simulink subsystem "SchlittenVorsteuerung"  (R2020a)
settings: Solver=VariableStepAuto  StartTime=0.0  StopTime=10.0  RelTol=1e-3
model mask{SP=simparams.gesamtmodell.schlittenpendel, vorst=simparams.vorst}
  mask prompts: SP "Schlitten Parameter"; vorst "Vorsteuerung"
undefined symbols (not defined in the file or in its folder): d0, Fc0, M, vorstC, vorstD, x0_p_c076_vorst
settings Model: Creator=Tobias  LastModifiedBy=Tobias

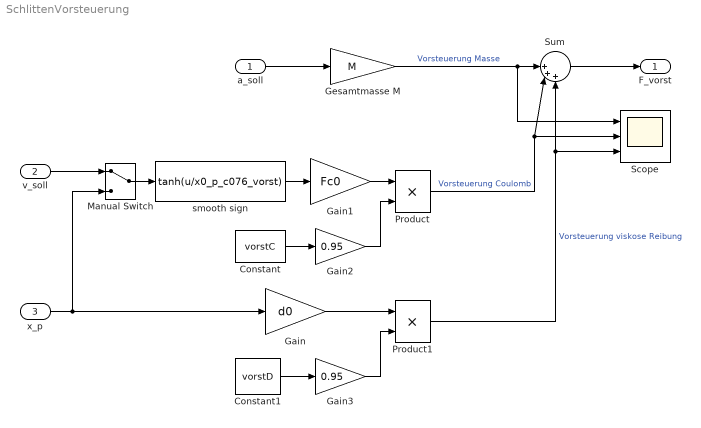
== system SchlittenVorsteuerung ==
  a_soll : Inport
  v_soll : Inport  Port=2
  x_p : Inport  Port=3
  Constant : Constant  Value=vorstC
  Constant1 : Constant  Value=vorstD
  Gain : Gain  Gain=d0
  Gain1 : Gain  Gain=Fc0
  Gain2 : Gain  Gain=0.95
  Gain3 : Gain  Gain=0.95
  Gesamtmasse M : Gain  Gain=M
  Manual Switch : ManualSwitch
  Product : Product  RndMeth=Zero
  Product1 : Product  RndMeth=Zero
  Scope : Scope  NumInputPorts=3
  Sum : Sum  Inputs=||+++
  smooth sign : Fcn  Expr=tanh(u/x0_p_c076_vorst)
  F_vorst : Outport
  wires:
  Constant1/1 -> Gain3/1
  Gain/1 -> Product1/1
  Product1/1 -> Scope/3, Sum/3  "Vorsteuerung viskose Reibung"
  x_p/1 -> Manual Switch/2, Gain/1
  Sum/1 -> F_vorst/1
  v_soll/1 -> Manual Switch/1
  a_soll/1 -> Gesamtmasse M/1
  Gain1/1 -> Product/1
  Gesamtmasse M/1 -> Scope/1, Sum/1  "Vorsteuerung Masse"
  Product/1 -> Scope/2, Sum/2  "Vorsteuerung Coulomb"
  Constant/1 -> Gain2/1
  smooth sign/1 -> Gain1/1
  Manual Switch/1 -> smooth sign/1
  Gain3/1 -> Product1/2
  Gain2/1 -> Product/2
